simulink model "nonlinear_plant"  (R2015a)
settings: Solver=ode45  StartTime=0.0  StopTime=100  RelTol=1e-3
undefined symbols (not defined in the file or in its folder): B, g, jp, l, mp
settings Model: Creator=morten  LastModifiedBy=morten
settings SolverCC: AlgebraicLoopSolver=LineSearch

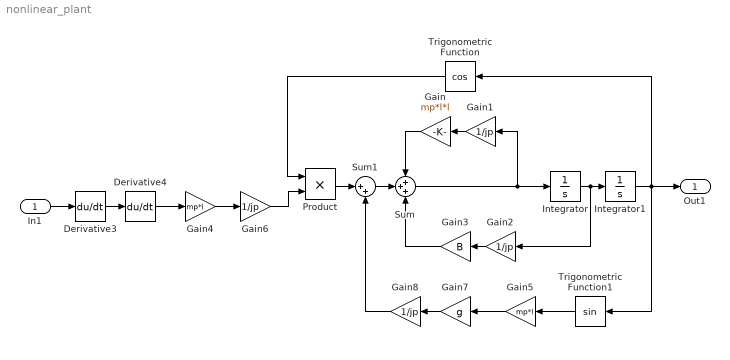
== system nonlinear_plant ==
  In1 : Inport
  Derivative3 : Derivative
  Derivative4 : Derivative
  Gain : Gain  Gain=mp*l*l
  Gain{1..2,6,8} (4 alike) : Gain  Gain=1/jp
  Gain3 : Gain  Gain=B
  Gain4 : Gain  Gain=mp*l
  Gain5 : Gain  Gain=mp*l
  Gain7 : Gain  Gain=g
  Integrator : Integrator
  Integrator1 : Integrator
  Product : Product
  Sum : Sum  Inputs=+++
  Sum1 : Sum  Inputs=|++
  Trigonometric Function : Trigonometry  Operator=cos
  Trigonometric Function1 : Trigonometry
  Out1 : Outport
  wires:
  Sum/1 -> Gain1/1, Integrator/1
  Integrator/1 -> Gain2/1, Integrator1/1
  Gain/1 -> Sum/1
  Gain1/1 -> Gain/1
  Gain2/1 -> Gain3/1
  Gain3/1 -> Sum/3
  Integrator1/1 -> Trigonometric Function1/1, Trigonometric Function/1, Out1/1
  In1/1 -> Derivative3/1
  Derivative3/1 -> Derivative4/1
  Derivative4/1 -> Gain4/1
  Product/1 -> Sum1/1
  Trigonometric Function/1 -> Product/1
  Gain4/1 -> Gain6/1
  Gain6/1 -> Product/2
  Trigonometric Function1/1 -> Gain5/1
  Gain5/1 -> Gain7/1
  Gain7/1 -> Gain8/1
  Gain8/1 -> Sum1/2
  Sum1/1 -> Sum/2
